simulink model "CoVM_TrqLeadCoord"  (R2016b)
settings: configuration reference "CodeGenConfigSet" (kept outside this file)
settings Model: Creator=Wollf  LastModifiedBy=bianxuyin
settings ConfigSetRef: SourceLocation=Base Workspace

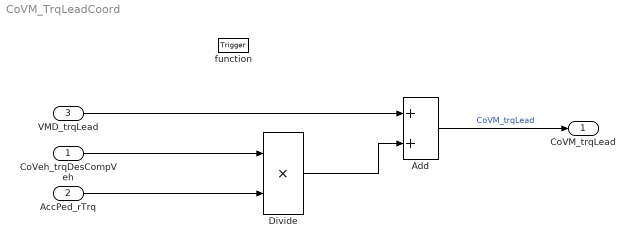
== system CoVM_TrqLeadCoord ==
  CoVeh_trqDesCompVeh : Inport  Tag=Nm  Description=Signal for compensation correction of wheel torque level (signal 1)  OutMin=-3000  OutMax=3000  OutDataTypeStr=Trq_Nm
  AccPed_rTrq : Inport  Description=Total drive train ratio of engine - wheel  Port=2  OutMin=-327  OutMax=327  OutDataTypeStr=TransRatio
  VMD_trqLead : Inport  Tag=Nm  Description=propulsion lead torque after driving assistance coordination  Port=3  OutMin=-3000  OutMax=3000  OutDataTypeStr=Trq_Nm
  function : TriggerPort  TriggerType=function-call  VariantControl=Variant
  Add : Sum  InputSameDT=on
  Divide : Product  Inputs=**  OutDataTypeStr=Trq_Nm  SaturateOnIntegerOverflow=on
  CoVM_trqLead : Outport  Tag=Nm  Description=Propulsion torque after coordination with ESP interventions(wheel torque)  OutMin=-3000  OutMax=3000  OutDataTypeStr=Trq_Nm
  wires:
  AccPed_rTrq/1 -> Divide/2
  Divide/1 -> Add/2
  VMD_trqLead/1 -> Add/1
  Add/1 -> CoVM_trqLead/1  "CoVM_trqLead"
  CoVeh_trqDesCompVeh/1 -> Divide/1
